simulink model "FixedWing_Model_nonlinearLQR_6_states"  (R2020b)
settings: Solver=VariableStepAuto  StartTime=0.0  StopTime=50  FixedStep=10^-4  RelTol=1e-7
values from neighbouring files (symbols this model uses):
  A_lat = [YB        Yp      -(u0-Yr)   g*cos(Theta0)   0;         A21       A22       A23        0             0;         A31       A32       A33        0             0;         0         1         0          0             0;         0         0         1          0             0]    [LQR_Dena_model_file_edited.m]
  A_long = [ Xu                    Xw              0              -g*cos(Theta0)            0;          Zu                    Zw              u0             -g*sin(Theta0)            0;          Mu+Mw_d*Zu            Mw+Mw_d*Zw      Mq+Mw_d*u0          0                    0;          0                     0               1                   0                    0;          -sin(Theta0)       -cos(Theta0)    ...(+51 chars)    [LQR_Dena_model_file_edited.m]
  b = 1.7    [LQR_Dena_model_file_edited.m]
  B_lat = [0        Ydr;        B21      B22;        B31      B32;        0        0;        0        0]    [LQR_Dena_model_file_edited.m]
  B_long = [ Xe         CXt;          Ze         0;          Me         0;          0          0;          0          0]    [LQR_Dena_model_file_edited.m]
  c = 0.28    [LQR_Dena_model_file_edited.m]
  C_lat = [0 0 0 1 0 ]    [LQR_Dena_model_file_edited.m]
  C_long = [0 0 0 1 0]    [LQR_Dena_model_file_edited.m]
  CL_aileron = 0.32935    [LQR_Dena_model_file_edited.m]
  CL_rudder = 0.003592    [LQR_Dena_model_file_edited.m]
  CLb = 0.029196    [LQR_Dena_model_file_edited.m]
  CLp = -0.44965    [LQR_Dena_model_file_edited.m]
  CLr = 0.0067709    [LQR_Dena_model_file_edited.m]
  CM_alpha = -0.1651    [LQR_Dena_model_file_edited.m]
  CM_alpha_dot = -6.5034    [LQR_Dena_model_file_edited.m]
  CMe = -1.3977    [LQR_Dena_model_file_edited.m]
  CMq = -11.7782    [LQR_Dena_model_file_edited.m]
  CMt = 0    [LQR_Dena_model_file_edited.m]
  CMu = 0.158*0    (= 0)    [LQR_Dena_model_file_edited.m]
  CN_aileron = 0.036215    [LQR_Dena_model_file_edited.m]
  CN_rudder = -0.045652    [LQR_Dena_model_file_edited.m]
  CNB = 0.066996    [LQR_Dena_model_file_edited.m]
  CNp = -0.030754    [LQR_Dena_model_file_edited.m]
  CNr = -0.064937    [LQR_Dena_model_file_edited.m]
  CX0 = -0.0094304    [LQR_Dena_model_file_edited.m]
  CX_alpha = (0.42565-0.21544)    (= 0.21021)    [LQR_Dena_model_file_edited.m]
  CXe = 0    [LQR_Dena_model_file_edited.m]
  CXt = 1    [LQR_Dena_model_file_edited.m]
  CXu = -(0.158*0)-0.0094304    (= -0.0094304)    [LQR_Dena_model_file_edited.m]
  CY_rudder = -0.10317    [LQR_Dena_model_file_edited.m]
  CYB = -0.16533    [LQR_Dena_model_file_edited.m]
  CYp = -0.00068802    [LQR_Dena_model_file_edited.m]
  CYr = 0.15502    [LQR_Dena_model_file_edited.m]
  CZ0 = -0.42565    [LQR_Dena_model_file_edited.m]
  CZ_alpha = -(4.8375+0.0094304)    (= -4.8469304)    [LQR_Dena_model_file_edited.m]
  CZ_alpha_dot = 1.3359    [LQR_Dena_model_file_edited.m]
  CZe = -0.56118    [LQR_Dena_model_file_edited.m]
  CZq = -7.3583    [LQR_Dena_model_file_edited.m]
  CZt = 0    [LQR_Dena_model_file_edited.m]
  CZu = -((0.052968^2)/(1-(0.052968)^2))*0.42565    (= -0.00119756738693)    [LQR_Dena_model_file_edited.m]
  d_aileron0 = 0    [LQR_Dena_model_file_edited.m]
  d_elevator0 = -0.6319*pi/180    (= -0.0110287355434)    [LQR_Dena_model_file_edited.m]
  D_long = zeros(5,2)    [LQR_Dena_model_file_edited.m]
  d_rudder0 = 0    [LQR_Dena_model_file_edited.m]
  d_Thrust0 = 5    [LQR_Dena_model_file_edited.m]
  e_longi = longd- [longi; 0]    [LQR_Dena_model_file_edited.m]
  Epsi0 = 0    [LQR_Dena_model_file_edited.m]
  Epsi_initial = Epsi0    (= 0)    [LQR_Dena_model_file_edited.m]
  g = 9.81    [LQR_Dena_model_file_edited.m]
  Hi = 120    [LQR_Dena_model_file_edited.m]
  Ix = 0.6465    [LQR_Dena_model_file_edited.m]
  Ixz = 0.0006584    [LQR_Dena_model_file_edited.m]
  Iy = 0.3048    [LQR_Dena_model_file_edited.m]
  Iz = 0.9359    [LQR_Dena_model_file_edited.m]
  K = K_long_hat(:,1:5)    [LQR_Dena_model_file_edited.m]
  K_lat_hat = lqr(A_lat_hat, B_lat_hat,Q_lat_hat,R_lat)    [LQR_Dena_model_file_edited.m]
  K_long = lqr(A_long, B_long,Q_long,R_long)    [LQR_Dena_model_file_edited.m]
  K_long_hat = lqr(A_long_hat, B_long_hat,Q_long_hat,R_long)    [LQR_Dena_model_file_edited.m]
  Ki = -K_long_hat(:,6)    [LQR_Dena_model_file_edited.m]
  lati = [ v_initial; p_initial; r_initial; Phi_initial; Epsi_initial]    [LQR_Dena_model_file_edited.m]
  longd = [u0; w0; q0; Theta0; Hi; 0]    [LQR_Dena_model_file_edited.m]
  longi = [ u_initial; w_initial; q_initial; Theta_initial; Ze0]    [LQR_Dena_model_file_edited.m]
  mass = 4    [LQR_Dena_model_file_edited.m]
  p0 = 0    [LQR_Dena_model_file_edited.m]
  p_initial = 0    [LQR_Dena_model_file_edited.m]
  Phi0 = 0    [LQR_Dena_model_file_edited.m]
  Phi_initial = Phi0    (= 0)    [LQR_Dena_model_file_edited.m]
  q0 = 0    [LQR_Dena_model_file_edited.m]
  q_initial = 0    [LQR_Dena_model_file_edited.m]
  r0 = 0    [LQR_Dena_model_file_edited.m]
  r_initial = 0    [LQR_Dena_model_file_edited.m]
  S = 0.471    [LQR_Dena_model_file_edited.m]
  Theta0 = 5.1*pi/180    (= 0.0890117918517)    [LQR_Dena_model_file_edited.m]
  Theta_initial = Theta0+(2*pi/180)    (= 0.123918376892)    [LQR_Dena_model_file_edited.m]
  u0 = sqrt(V0^2/(1+(tan(Theta0))^2))    [LQR_Dena_model_file_edited.m]
  u_initial = u0    [LQR_Dena_model_file_edited.m]
  v0 = 0    [LQR_Dena_model_file_edited.m]
  v_initial = v0    (= 0)    [LQR_Dena_model_file_edited.m]
  w0 = u0*tan(Theta0)    [LQR_Dena_model_file_edited.m]
  w_initial = w0    [LQR_Dena_model_file_edited.m]
  X0 = mass*g*sin(Theta0)    [LQR_Dena_model_file_edited.m]
  Xe0 = 0    [LQR_Dena_model_file_edited.m]
  Y0 = -mass*g*cos(Theta0)*sin(Phi0)    [LQR_Dena_model_file_edited.m]
  Ye0 = 0    [LQR_Dena_model_file_edited.m]
  Z0 = -mass*g*cos(Theta0)*cos(Phi0)    [LQR_Dena_model_file_edited.m]
  Ze0 = 120    [LQR_Dena_model_file_edited.m]
undefined symbols (not defined in the file or in its folder): A_hat, B_hat, C_hat, K_alt, K_e, Meu_e, use, W_e
libraries: simulink_extras x39, dspindex x3, aerolibatmos2 x1, aerolibutil x1, sharedtransform x1
(part 1 of 2)
settings Model: Creator=IT Solutions  LastModifiedBy=Roooooomaaaaaaaaaaaa
settings SolverCC: AlgebraicLoopSolver=LineSearch
settings DebuggingCC: UnconnectedInputMsg=none  UnconnectedOutputMsg=none  UnconnectedLineMsg=none  SFMachineParentedDataDiag=error

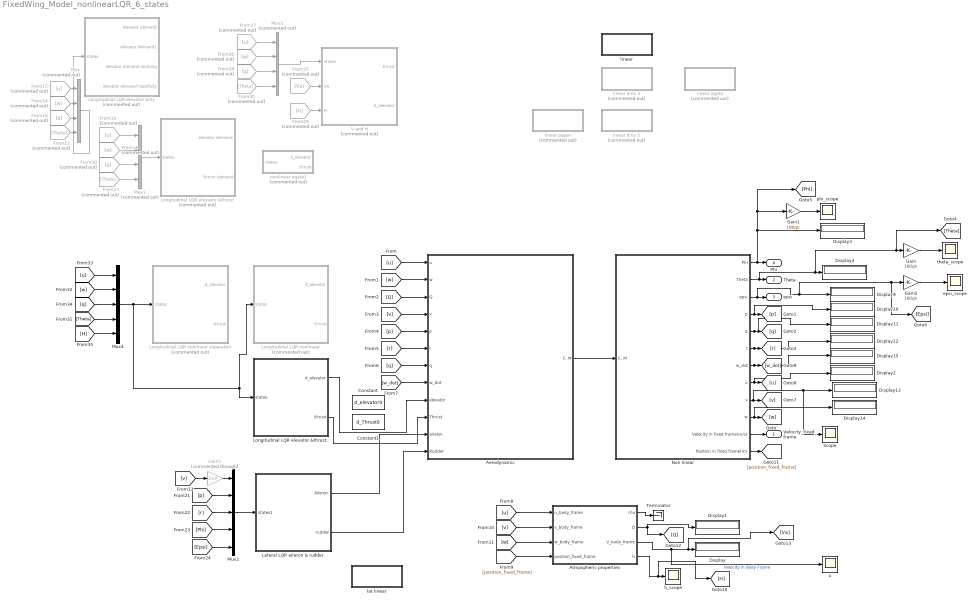
== system FixedWing_Model_nonlinearLQR_6_states ==
  "Aerodynamic " : Subsystem
  Atmpspheric properties : Subsystem
  Constant : Constant  Value=d_elevator0
  Constant1 : Constant  Value=d_Thrust0
  Display{,1..4,9..15} (12 alike) : Display
  From12 : From  Commented=on  GotoTag=Theta
  From14 : From  Commented=on  GotoTag=w
  From15 : From  Commented=on  GotoTag=u
  From16 : From  Commented=on  GotoTag=q
  From17 : From  Commented=on  GotoTag=Theta
  From18 : From  Commented=on  GotoTag=w
  From19 : From  Commented=on  GotoTag=u
  From20 : From  Commented=on  GotoTag=q
  From25 : From  Commented=on  GotoTag=Va
  From26 : From  Commented=on  GotoTag=w
  From27 : From  Commented=on  GotoTag=u
  From28 : From  Commented=on  GotoTag=q
  From29 : From  Commented=on  GotoTag=H
  From30 : From  Commented=on  GotoTag=Theta
  Gain : Gain  Gain=180/pi
  Gain1 : Gain  Gain=180/pi
  Gain2 : Gain  Gain=180/pi
  Gain3 : Gain  Commented=through  Gain=1/u0
  Lateral LQR aileron & rudder : Subsystem
  Longitudinal LQR elevator &thrust : Subsystem  Commented=on
  Longitudinal LQR elevator &thrust. : Subsystem
  Longitudinal LQR elevator only : Subsystem  Commented=on
  Longitudinal LQR nonlinear : Subsystem  Commented=on
  Longitudinal LQR nonlinear seperated : Subsystem  Commented=on
  Mux : Mux  Commented=on
  Mux1 : Mux  Commented=on
  Mux2 : Mux  Inputs=5
  Mux3 : Mux  Commented=on
  Mux4 : Mux  Inputs=5
  Non linear : Subsystem
  Scope : Scope
  Terminator : Terminator
  V and H : Subsystem  Commented=on
  epsi_scope : Scope
  h_scope : Scope
  lat linear : Subsystem
  linear : Subsystem
  linear dina 4 : Subsystem  Commented=on
  linear dina 5 : Subsystem  Commented=on
  linear ogata : Subsystem  Commented=on
  linear paper : Subsystem  Commented=on
  nonlinear ogata1 : Subsystem  Commented=on
  phi_scope : Scope
  theta_scope : Scope
  u : Scope
  Velocity_fixed_frame : Outport
  Theta : Outport  Port=2
  epsi : Outport  Port=3
  Phi : Outport  Port=4
  wires:
  [u] -> "Aerodynamic "/1(u)
  [w] -> "Aerodynamic "/2(w)
  [v] -> "Aerodynamic "/4(v)
  [p] -> "Aerodynamic "/5(p)
  [r] -> "Aerodynamic "/6(r)
  [q] -> "Aerodynamic "/7(q)
  [w_dot] -> "Aerodynamic "/8(w_dot)
  Non linear/4(p) -> Display10/1, [p]
  Non linear/5(q) -> Display11/1, [q]
  Non linear/6(r) -> Display12/1, [r]
  Non linear/1(Phi) -> Display3/1, Gain1/1, [Phi], Phi/1
  Non linear/3(epsi) -> Gain2/1, [Epsi], Display9/1, epsi/1
  Non linear/7(w_dot) -> Display15/1, [w_dot]
  Non linear/8(u) -> Display2/1, [u]
  Non linear/9(v) -> Scope/1, Display13/1, [v]
  Non linear/10(w) -> Display14/1, [w]
  Non linear/11(Velocity in fixed frame(m/s)) -> Velocity_fixed_frame/1
  Non linear/12(Position in fixed frame(m)) -> [position_fixed_frame]
  [position_fixed_frame] -> Atmpspheric properties/4(position_fixed_frame)
  Atmpspheric properties/2(Q) -> [Q], Display1/1
  Atmpspheric properties/1(rho) -> Terminator/1
  [u] -> Atmpspheric properties/1(u_body_frame)
  [v] -> Atmpspheric properties/2(v_body_frame)
  [w] -> Atmpspheric properties/3(w_body_frame)
  Atmpspheric properties/3(V_body_frame) -> u/1, [Va], Display/1  "Velocity in Body Frame"
  Non linear/2(Theta) -> [Theta], Gain/1, Display4/1, Theta/1
  [Q] -> "Aerodynamic "/3(Q)
  "Aerodynamic "/1("F, M") -> Non linear/1("F, M")
  Gain/1 -> theta_scope/1
  Atmpspheric properties/4(h) -> [H], h_scope/1
  Gain1/1 -> phi_scope/1
  Gain2/1 -> epsi_scope/1
  From12/1 -> Mux/4
  From16/1 -> Mux/3
  From14/1 -> Mux/2
  From15/1 -> Mux/1
  Mux/1 -> Longitudinal LQR elevator only/1(states)
  From20/1 -> Mux1/3
  From17/1 -> Mux1/4
  Mux1/1 -> Longitudinal LQR elevator &thrust/1(states)
  From18/1 -> Mux1/2
  From19/1 -> Mux1/1
  Mux2/1 -> Lateral LQR aileron & rudder/1(states1)
  [p] -> Mux2/2
  [r] -> Mux2/3
  [Phi] -> Mux2/4
  [v] -> Gain3/1
  From26/1 -> Mux3/2
  From30/1 -> Mux3/4
  From27/1 -> Mux3/1
  From28/1 -> Mux3/3
  Mux3/1 -> V and H/1(states)
  From25/1 -> V and H/2(Va)
  From29/1 -> V and H/3(H)
  [w] -> Mux4/2
  [Theta] -> Mux4/4
  [q] -> Mux4/3
  [u] -> Mux4/1
  Mux4/1 -> Longitudinal LQR nonlinear/1(states), Longitudinal LQR elevator &thrust./1(states), Longitudinal LQR nonlinear seperated/1(states)
  [H] -> Mux4/5
  Lateral LQR aileron & rudder/1(Aileron) -> "Aerodynamic "/11(airelon)
  Lateral LQR aileron & rudder/2(rudder) -> "Aerodynamic "/12(Rudder)
  [Epsi] -> Mux2/5
  Gain3/1 -> Mux2/1
  Longitudinal LQR elevator &thrust./1(d_elevator) -> "Aerodynamic "/9(elevator)
  Longitudinal LQR elevator &thrust./2(thrust) -> "Aerodynamic "/10(Thrust)

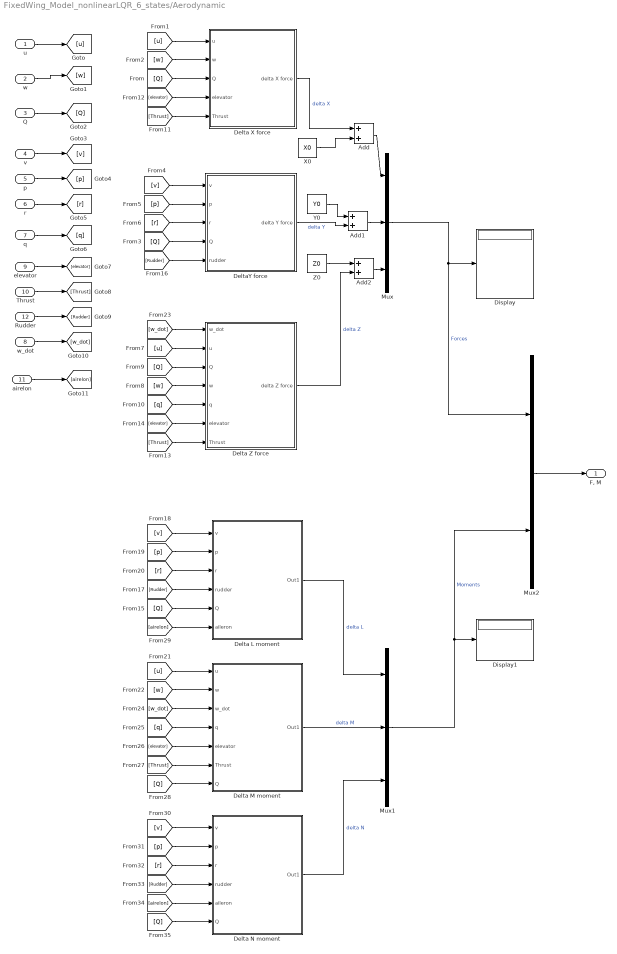
== system FixedWing_Model_nonlinearLQR_6_states/Aerodynamic  ==
  u : Inport
  w : Inport  Port=2
  Q : Inport  Port=3
  v : Inport  Port=4
  p : Inport  Port=5
  r : Inport  Port=6
  q : Inport  Port=7
  w_dot : Inport  Port=8
  elevator : Inport  Port=9
  Thrust : Inport  Port=10
  airelon : Inport  Port=11
  Rudder : Inport  Port=12
  Add : Sum
  Add1 : Sum
  Add2 : Sum
  Delta L moment : Subsystem
  Delta M moment : Subsystem
  Delta N moment : Subsystem
  Delta X force : Subsystem
  Delta Z force : Subsystem
  DeltaY force : Subsystem
  Display : Display
      settings: Decimation=3
  Display1 : Display
      settings: Decimation=3
  Mux : Mux  Inputs=3
  Mux1 : Mux  Inputs=3
  Mux2 : Mux  Inputs=2
  X0 : Constant  Value=X0
  Y0 : Constant  Value=Y0
  Z0 : Constant  Value=Z0
  "F, M" : Outport
  wires:
  Mux/1 -> Mux2/1, Display/1  "Forces"
  Mux1/1 -> Mux2/2, Display1/1  "Moments"
  DeltaY force/1(delta Y force) -> Add1/2  "delta Y"
  Delta L moment/1(Out1) -> Mux1/1  "delta L"
  Mux2/1 -> "F, M"/1
  Q/1 -> [Q]
  w/1 -> [w]
  u/1 -> [u]
  Delta N moment/1(Out1) -> Mux1/3  "delta N"
  [Q] -> DeltaY force/4(Q)
  [Rudder] -> DeltaY force/5(rudder)
  v/1 -> [v]
  p/1 -> [p]
  r/1 -> [r]
  [v] -> DeltaY force/1(v)
  [p] -> DeltaY force/2(p)
  [r] -> DeltaY force/3(r)
  q/1 -> [q]
  elevator/1 -> [elevator]
  Thrust/1 -> [Thrust]
  [Q] -> Delta L moment/5(Q)
  Rudder/1 -> [Rudder]
  [Rudder] -> Delta L moment/4(rudder)
  [v] -> Delta L moment/1(v)
  [p] -> Delta L moment/2(p)
  [r] -> Delta L moment/3(r)
  w_dot/1 -> [w_dot]
  airelon/1 -> [airelon]
  [airelon] -> Delta L moment/6(aileron)
  [v] -> Delta N moment/1(v)
  [p] -> Delta N moment/2(p)
  [r] -> Delta N moment/3(r)
  [Rudder] -> Delta N moment/4(rudder)
  [airelon] -> Delta N moment/5(aileron)
  [Q] -> Delta N moment/6(Q)
  X0/1 -> Add/2
  Y0/1 -> Add1/1
  Z0/1 -> Add2/1
  Add/1 -> Mux/1
  Add1/1 -> Mux/2
  Add2/1 -> Mux/3
  [u] -> Delta Z force/2(u)
  [w] -> Delta Z force/4(w)
  [w_dot] -> Delta Z force/1(w_dot)
  Delta Z force/1(delta Z force) -> Add2/2  "delta Z"
  [Q] -> Delta Z force/3(Q)
  [q] -> Delta Z force/5(q)
  [elevator] -> Delta Z force/6(elevator)
  [w] -> Delta X force/2(w)
  [elevator] -> Delta X force/4(elevator)
  [Q] -> Delta X force/3(Q)
  [u] -> Delta X force/1(u)
  Delta X force/1(delta X force) -> Add/1  "delta X"
  [q] -> Delta M moment/4(q)
  Delta M moment/1(Out1) -> Mux1/2  "delta M"
  [elevator] -> Delta M moment/5(elevator)
  [Q] -> Delta M moment/7(Q)
  [Thrust] -> Delta M moment/6(Thrust)
  [w] -> Delta M moment/2(w)
  [w_dot] -> Delta M moment/3(w_dot)
  [u] -> Delta M moment/1(u)
  [Thrust] -> Delta X force/5(Thrust)
  [Thrust] -> Delta Z force/7(Thrust)

== system FixedWing_Model_nonlinearLQR_6_states/Atmpspheric properties ==
  u_body_frame : Inport
  v_body_frame : Inport  Port=2
  w_body_frame : Inport  Port=3
  position_fixed_frame : Inport  Port=4
  Add : Sum  Inputs=+++
  Demux : Demux  Outputs=3
  Display : Display
  Gain : Gain  Gain=1/2
  ISA Atmosphere Model : aerolibatmos2/ISA Atmosphere Model  custom=off  g=9.80665  gamma=1.4  R=287.0531  L=0.0065  h_trop=11000  h_strat=20000  rho0=1.225  P0=101325  T0=288.15  h0=0
  Product : Product
  Scope : Scope
  Sqrt : Sqrt  SaturateOnIntegerOverflow=on
  Square : Math  Operator=square  SaturateOnIntegerOverflow=on
  Square1 : Math  Operator=square  SaturateOnIntegerOverflow=on
  Square2 : Math  Operator=square  SaturateOnIntegerOverflow=on
  Terminator : Terminator
  Terminator1 : Terminator
  rho : Outport
  Q : Outport  Port=2
  V_body_frame : Outport  Port=3
  h : Outport  Port=4
  wires:
  position_fixed_frame/1 -> Demux/1
  Demux/1 -> Terminator/1
  Demux/2 -> Terminator1/1
  Demux/3 -> Scope/1, h/1, ISA Atmosphere Model/1
  ISA Atmosphere Model/4 -> [rho], rho/1
  Square/1 -> Add/1
  Square1/1 -> Add/2
  Square2/1 -> Add/3
  Add/1 -> Sqrt/1, Gain/1
  Gain/1 -> Product/2
  [rho] -> Product/1
  Product/1 -> Q/1
  u_body_frame/1 -> Square/1
  v_body_frame/1 -> Square1/1
  w_body_frame/1 -> Square2/1
  Sqrt/1 -> Display/1, V_body_frame/1

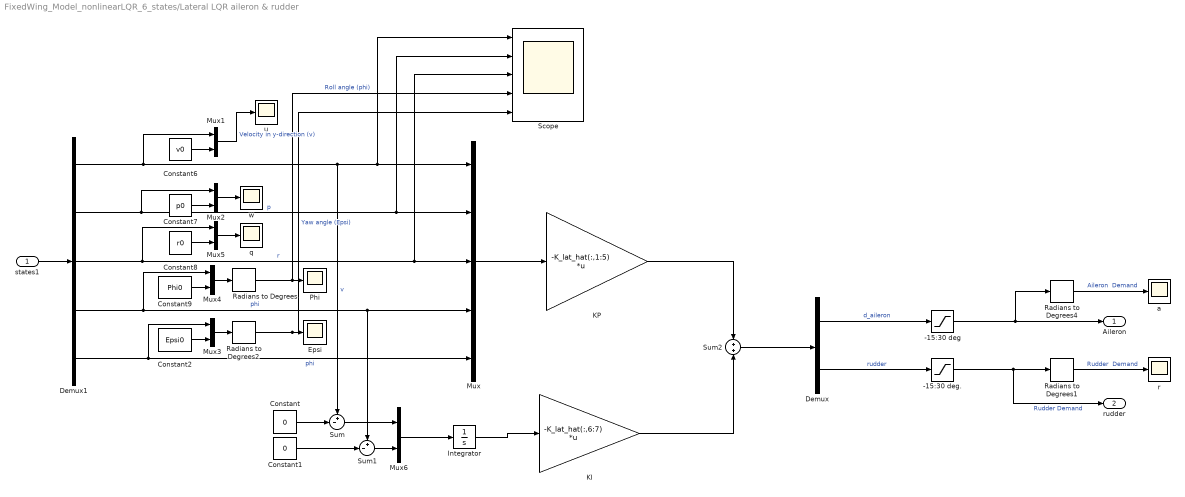
== system FixedWing_Model_nonlinearLQR_6_states/Lateral LQR aileron & rudder ==
  states1 : Inport
  -15:30 deg : Saturate  UpperLimit=30*pi/180  LowerLimit=-15*pi/180
  -15:30 deg. : Saturate  UpperLimit=30*pi/180  LowerLimit=-15*pi/180
  Constant : Constant  Value=0
  Constant1 : Constant  Value=0
  Constant2 : Constant  Value=Epsi0
  Constant6 : Constant  Value=v0
  Constant7 : Constant  Value=p0
  Constant8 : Constant  Value=r0
  Constant9 : Constant  Value=Phi0
  Demux : Demux  Outputs=2
  Demux1 : Demux  Outputs=5
  Epsi : Scope
  Integrator : Integrator
  KI : Gain  Gain=-K_lat_hat(:,6:7)  Multiplication=Matrix(K*u)
  KP : Gain  Gain=-K_lat_hat(:,1:5)  Multiplication=Matrix(K*u)
  Mux : Mux  Inputs=5
  Mux{1..6} (6 alike) : Mux  Inputs=2
  Phi : Scope
  Radians to Degrees{,1..2,4} (4 alike) : simulink_extras/Transformations/Radians to Degrees
  Scope : Scope  NumInputPorts=5
  Sum : Sum  Inputs=+-|
  Sum1 : Sum  Inputs=+-|
  Sum2 : Sum  Inputs=+|+
  a : Scope
  q : Scope
  r : Scope
  u : Scope
  w : Scope
  Aileron : Outport
  rudder : Outport  Port=2
  wires:
  Sum2/1 -> Demux/1
  Demux1/2 -> Scope/2, Mux/2, Mux2/1  "p"
  Constant9/1 -> Mux4/2
  Mux1/1 -> u/1  "Velocity in y-direction (v)"
  Constant/1 -> Sum/2
  Mux/1 -> KP/1
  Demux1/4 -> Mux4/1, Sum1/1, Mux/4  "phi"
  Constant6/1 -> Mux1/2
  Integrator/1 -> KI/1
  KP/1 -> Sum2/1
  Mux4/1 -> Radians to Degrees/1
  Mux6/1 -> Integrator/1
  Sum1/1 -> Mux6/2
  Mux5/1 -> q/1
  Sum/1 -> Mux6/1
  Constant8/1 -> Mux5/2
  Demux1/1 -> Scope/1, Mux/1, Sum/1, Mux1/1  "v"
  Constant7/1 -> Mux2/2
  KI/1 -> Sum2/2
  Radians to Degrees/1 -> Scope/4, Phi/1  "Roll angle (phi)"
  Mux2/1 -> w/1
  Radians to Degrees4/1 -> a/1  "Aileron  Demand"
  Demux/2 -> -15:30 deg./1  "rudder"
  Demux/1 -> -15:30 deg/1  "d_aileron"
  states1/1 -> Demux1/1
  Constant1/1 -> Sum1/2
  -15:30 deg/1 -> Radians to Degrees4/1, Aileron/1
  Demux1/3 -> Scope/3, Mux/3, Mux5/1  "r"
  -15:30 deg./1 -> Radians to Degrees1/1, rudder/1  "Rudder Demand"
  Radians to Degrees1/1 -> r/1  "Rudder  Demand"
  Radians to Degrees2/1 -> Scope/5, Epsi/1  "Yaw angle (Epsi)"
  Mux3/1 -> Radians to Degrees2/1
  Demux1/5 -> Mux3/1, Mux/5  "phi"
  Constant2/1 -> Mux3/2

== system FixedWing_Model_nonlinearLQR_6_states/Longitudinal LQR elevator &thrust ==
  states : Inport
  all system : Subsystem
  "elevator demand " : Outport
  thrust demand : Outport  Port=2
  wires:
  all system/1(d_elevator) -> "elevator demand "/1
  states/1 -> all system/1(states)
  all system/2(thrust) -> thrust demand/1

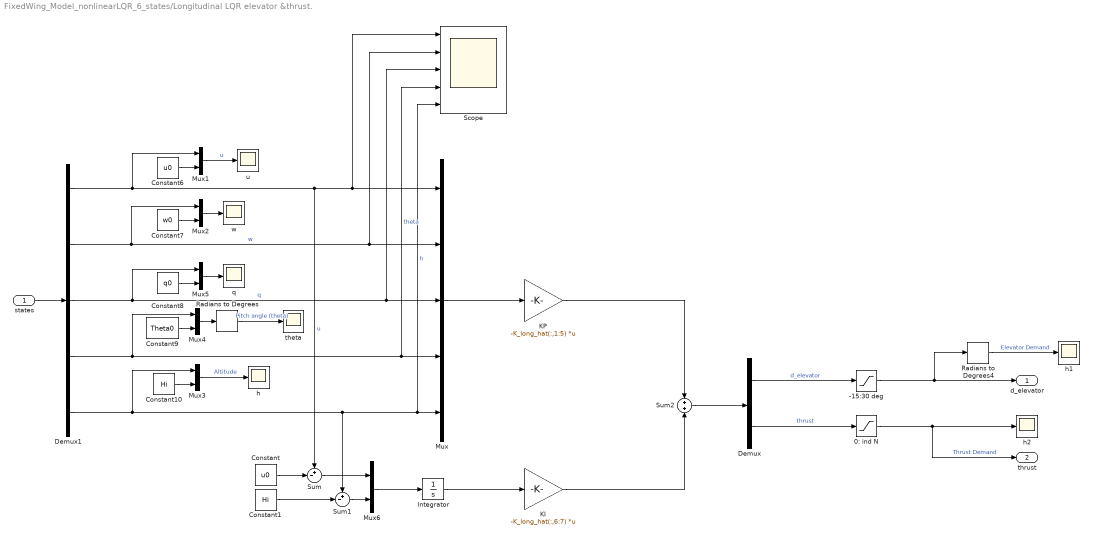
== system FixedWing_Model_nonlinearLQR_6_states/Longitudinal LQR elevator &thrust. ==
  states : Inport
  -15:30 deg : Saturate  UpperLimit=30*pi/180  LowerLimit=-15*pi/180
  0: ind N : Saturate  UpperLimit=inf  LowerLimit=0
  Constant : Constant  Value=u0
  Constant1 : Constant  Value=Hi
  Constant10 : Constant  Value=Hi
  Constant6 : Constant  Value=u0
  Constant7 : Constant  Value=w0
  Constant8 : Constant  Value=q0
  Constant9 : Constant  Value=Theta0
  Demux : Demux  Outputs=2
  Demux1 : Demux  Outputs=5
  Integrator : Integrator
  KI : Gain  Gain=-K_long_hat(:,6:7)  Multiplication=Matrix(K*u)
  KP : Gain  Gain=-K_long_hat(:,1:5)  Multiplication=Matrix(K*u)
  Mux : Mux  Inputs=5
  Mux{1..6} (6 alike) : Mux  Inputs=2
  Radians to Degrees : simulink_extras/Transformations/Radians to Degrees
  Radians to Degrees4 : simulink_extras/Transformations/Radians to Degrees
  Scope : Scope  NumInputPorts=5
  Sum : Sum  Inputs=+-|
  Sum1 : Sum  Inputs=+-|
  Sum2 : Sum  Inputs=+|+
  h : Scope
  h1 : Scope
  h2 : Scope
  q : Scope
  theta : Scope
  u : Scope
  w : Scope
  d_elevator : Outport
  thrust : Outport  Port=2
  wires:
  Radians to Degrees4/1 -> h1/1  "Elevator Demand"
  Demux/2 -> 0: ind N/1  "thrust"
  Demux/1 -> -15:30 deg/1  "d_elevator"
  KP/1 -> Sum2/1
  -15:30 deg/1 -> Radians to Degrees4/1, d_elevator/1
  0: ind N/1 -> h2/1, thrust/1  "Thrust Demand"
  states/1 -> Demux1/1
  Mux5/1 -> q/1
  Sum/1 -> Mux6/1
  Sum1/1 -> Mux6/2
  Demux1/5 -> Scope/5, Mux/5, Sum1/1, Mux3/1  "h"
  Mux4/1 -> Radians to Degrees/1
  Mux6/1 -> Integrator/1
  Constant6/1 -> Mux1/2
  Integrator/1 -> KI/1
  Demux1/4 -> Scope/4, Mux/4, Mux4/1  "theta"
  Mux/1 -> KP/1
  Mux2/1 -> w/1
  Demux1/3 -> Scope/3, Mux/3, Mux5/1  "q"
  Constant/1 -> Sum/2
  Mux1/1 -> u/1  "u"
  Constant10/1 -> Mux3/2
  Constant9/1 -> Mux4/2
  Radians to Degrees/1 -> theta/1  "Pitch angle (theta)"
  Demux1/2 -> Scope/2, Mux/2, Mux2/1  "w"
  Demux1/1 -> Scope/1, Mux/1, Sum/1, Mux1/1  "u"
  KI/1 -> Sum2/2
  Constant7/1 -> Mux2/2
  Mux3/1 -> h/1  "Altitude"
  Constant1/1 -> Sum1/2
  Constant8/1 -> Mux5/2
  Sum2/1 -> Demux/1

== system FixedWing_Model_nonlinearLQR_6_states/Longitudinal LQR elevator only ==
  states : Inport
  Actual theta2 : Scope
  Demux1 : Demux
  Radians to Degrees6 : simulink_extras/Transformations/Radians to Degrees
  Servo2 : TransferFcn  Commented=on  Numerator=[K_e]  Denominator=[W_e^(-2) (2*Meu_e/W_e) 1]
  all system : Subsystem
  states from ss : Subsystem  Commented=on
  theta from ss : Subsystem  Commented=on
  theta system only : Subsystem
  elevator demand : Outport
  elevator demand1 : Outport  Port=2
  elevator demand working : Outport  Port=3
  elevator demand hopefully : Outport  Port=4
  wires:
  Radians to Degrees6/1 -> Actual theta2/1
  Demux1/4 -> Radians to Degrees6/1, [theta]
  theta system only/1(d_elevator) -> elevator demand working/1
  [theta] -> theta system only/1(theta)
  all system/1(d_elevator) -> elevator demand hopefully/1
  states/1 -> Demux1/1, all system/1(states)
  theta from ss/1(elevator demand) -> elevator demand/1
  states from ss/1(elevator demand1) -> elevator demand1/1

== system FixedWing_Model_nonlinearLQR_6_states/Longitudinal LQR nonlinear ==
  states : Inport
  Constant1 : Constant  Value=d_elevator0
  Constant2 : Constant  Value=d_Thrust0
  Demux : Demux  Outputs=2
  Gain : Gain
  Gain1 : Gain
  K_LQR : Gain  Gain=K_long_hat  Multiplication=Matrix(K*u)
  Radians to Degrees4 : simulink_extras/Transformations/Radians to Degrees
  Sum1 : Sum  Inputs=|++
  Sum2 : Sum  Inputs=|++
  Thrust : Scope
  elevator2 : Scope
  states' error : Subsystem
  d_elevator : Outport
  thrust : Outport  Port=2
  wires:
  Demux/2 -> Sum2/1
  Demux/1 -> Sum1/1
  Sum2/1 -> Gain1/1, Thrust/1  "thrust"
  Sum1/1 -> Gain/1, Radians to Degrees4/1  "d_elevator"
  states' error/1(states' error) -> K_LQR/1
  Radians to Degrees4/1 -> elevator2/1
  states/1 -> states' error/1(In1)
  K_LQR/1 -> Demux/1
  Constant1/1 -> Sum1/2
  Constant2/1 -> Sum2/2
  Gain/1 -> d_elevator/1
  Gain1/1 -> thrust/1

== system FixedWing_Model_nonlinearLQR_6_states/Longitudinal LQR nonlinear seperated ==
  states : Inport
  Constant1 : Constant  Value=d_elevator0
  Constant2 : Constant  Value=d_Thrust0
  Demux : Demux  Outputs=2
  Gain : Gain  Gain=K  Multiplication=Matrix(K*u)
  Gain1 : Gain  Gain=Ki  Multiplication=Matrix(K*u)
  Integrator : Integrator
  Radians to Degrees4 : simulink_extras/Transformations/Radians to Degrees
  Sum1 : Sum  Inputs=|++
  Sum2 : Sum  Inputs=|++
  Sum3 : Sum  Inputs=|-+
  Thrust : Scope
  elevator2 : Scope
  theta' error : Subsystem
  d_elevator : Outport
  thrust : Outport  Port=2
  wires:
  Demux/2 -> Sum2/1
  Demux/1 -> Sum1/1
  Sum2/1 -> thrust/1, Thrust/1  "thrust"
  Sum1/1 -> d_elevator/1, Radians to Degrees4/1  "d_elevator"
  Radians to Degrees4/1 -> elevator2/1
  states/1 -> Gain/1, theta' error/1(states)
  Constant1/1 -> Sum1/2
  Constant2/1 -> Sum2/2
  Gain/1 -> Sum3/1
  Integrator/1 -> Gain1/1
  Gain1/1 -> Sum3/2
  theta' error/1(theta' error) -> Integrator/1
  Sum3/1 -> Demux/1  "d_elevator"

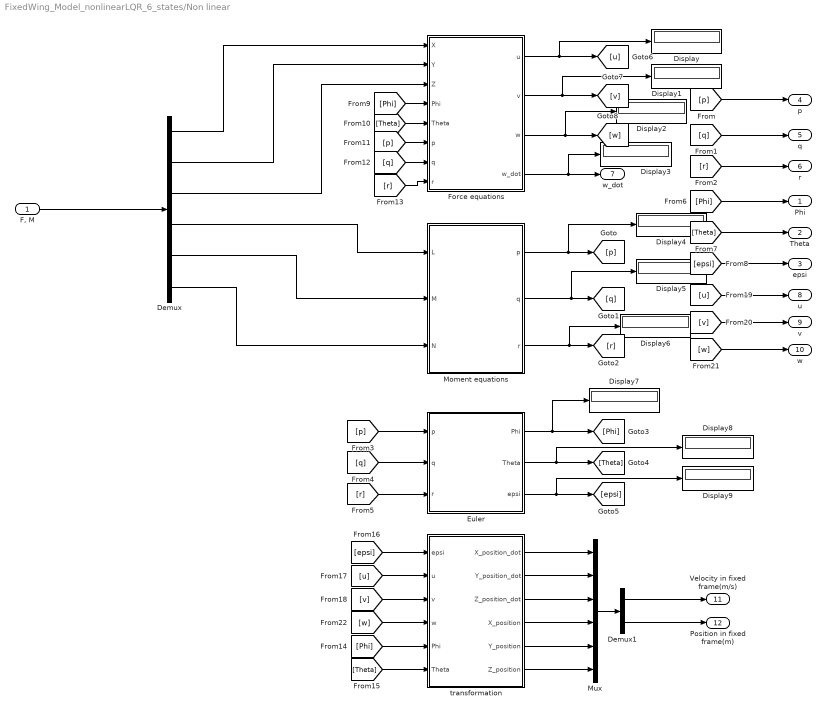
== system FixedWing_Model_nonlinearLQR_6_states/Non linear ==
  "F, M" : Inport
  Demux : Demux  Outputs=6
  Demux1 : Demux  Outputs=2
  Display{,1..9} (10 alike) : Display
  Euler : Subsystem
  Force equations : Subsystem
  Moment equations : Subsystem
  Mux : Mux  Inputs=6
  transformation : Subsystem
  Phi : Outport
  Theta : Outport  Port=2
  epsi : Outport  Port=3
  p : Outport  Port=4
  q : Outport  Port=5
  r : Outport  Port=6
  w_dot : Outport  Port=7
  u : Outport  Port=8
  v : Outport  Port=9
  w : Outport  Port=10
  Velocity in fixed frame(m/s) : Outport  Port=11
  Position in fixed frame(m) : Outport  Port=12
  wires:
  "F, M"/1 -> Demux/1
  Demux/2 -> Force equations/2(Y)
  Demux/4 -> Moment equations/1(L)
  Demux/3 -> Force equations/3(Z)
  Demux/1 -> Force equations/1(X)
  Force equations/1(u) -> Display/1, [u]
  Force equations/2(v) -> Display1/1, [v]
  Force equations/3(w) -> Display2/1, [w]
  [p] -> p/1
  [r] -> r/1
  [q] -> q/1
  Moment equations/2(q) -> Display5/1, [q]
  Moment equations/1(p) -> Display4/1, [p]
  Moment equations/3(r) -> Display6/1, [r]
  Demux/5 -> Moment equations/2(M)
  Demux/6 -> Moment equations/3(N)
  [q] -> Euler/2(q)
  [p] -> Euler/1(p)
  [r] -> Euler/3(r)
  [Phi] -> Phi/1
  [Theta] -> Theta/1
  [epsi] -> epsi/1
  Euler/1(Phi) -> Display7/1, [Phi]
  Euler/2(Theta) -> Display8/1, [Theta]
  Euler/3(epsi) -> Display9/1, [epsi]
  [Phi] -> Force equations/4(Phi)
  [Theta] -> Force equations/5(Theta)
  [p] -> Force equations/6(p)
  [q] -> Force equations/7(q)
  [r] -> Force equations/8(r)
  Force equations/4(w_dot) -> Display3/1, w_dot/1
  [u] -> u/1
  [v] -> v/1
  [w] -> w/1
  [Theta] -> transformation/6(Theta)
  [v] -> transformation/3(v)
  [u] -> transformation/2(u)
  [Phi] -> transformation/5(Phi)
  [epsi] -> transformation/1(epsi)
  [w] -> transformation/4(w)
  transformation/1(X_position_dot) -> Mux/1
  transformation/2(Y_position_dot) -> Mux/2
  transformation/3(Z_position_dot) -> Mux/3
  transformation/4(X_position) -> Mux/4
  transformation/5(Y_position) -> Mux/5
  transformation/6(Z_position) -> Mux/6
  Mux/1 -> Demux1/1
  Demux1/1 -> Velocity in fixed frame(m/s)/1
  Demux1/2 -> Position in fixed frame(m)/1

== system FixedWing_Model_nonlinearLQR_6_states/V and H ==
  states : Inport
  Va : Inport  Port=2
  H : Inport  Port=3
  Actual theta : Scope
  Constant : Constant  Value=120
  Constant1 : Constant  Value=d_elevator0
  Constant2 : Constant  Value=d_Thrust0
  Constant3 : Constant  Value=0
  Constant4 : Constant  Value=0
  Constant5 : Constant  Value=K_alt
  Demux : Demux  Outputs=2
  Derivative : Derivative
  Derivative1 : Derivative
  Gain1 : Gain
  Gain2 : Gain
  K_LQR : Gain  Gain=K_long  Multiplication=Matrix(K*u)
  MatrixMultiply : Product  Inputs=**  Multiplication=Matrix(*)
  Mux : Mux  Inputs=3
  Radians to Degrees4 : simulink_extras/Transformations/Radians to Degrees
  Sum1 : Sum  Inputs=|++
  Sum2 : Sum  Inputs=|++
  Sum3 : Sum  Inputs=|-+
  Sum4 : Sum  Inputs=|-+
  Sum5 : Sum  Inputs=|-+
  Thrust : Scope
  elevator2 : Scope
  states' error : Subsystem
  thrust : Outport
  d_elevator : Outport  Port=2
  wires:
  states' error/1(theta in degrees) -> Actual theta/1
  Gain1/1 -> thrust/1  "thrust"
  Sum2/1 -> Thrust/1, Gain1/1
  Demux/2 -> Sum2/1
  states/1 -> states' error/1(In1)
  states' error/2(states' error) -> K_LQR/1
  Constant2/1 -> Sum2/2
  K_LQR/1 -> Demux/1
  Constant1/1 -> Sum1/2
  Sum1/1 -> Gain2/1, Radians to Degrees4/1
  MatrixMultiply/1 -> Sum1/1
  Gain2/1 -> d_elevator/1  "d_elevator"
  Radians to Degrees4/1 -> elevator2/1
  Constant/1 -> Sum5/2
  H/1 -> Derivative/1, Sum5/1
  Derivative/1 -> Sum3/1, Derivative1/1
  Constant3/1 -> Sum3/2
  Constant4/1 -> Sum4/2
  Derivative1/1 -> Sum4/1
  Sum5/1 -> Mux/1  "error q"
  Sum3/1 -> Mux/2  "error q"
  Sum4/1 -> Mux/3  "error q"
  Mux/1 -> MatrixMultiply/1
  Constant5/1 -> MatrixMultiply/2

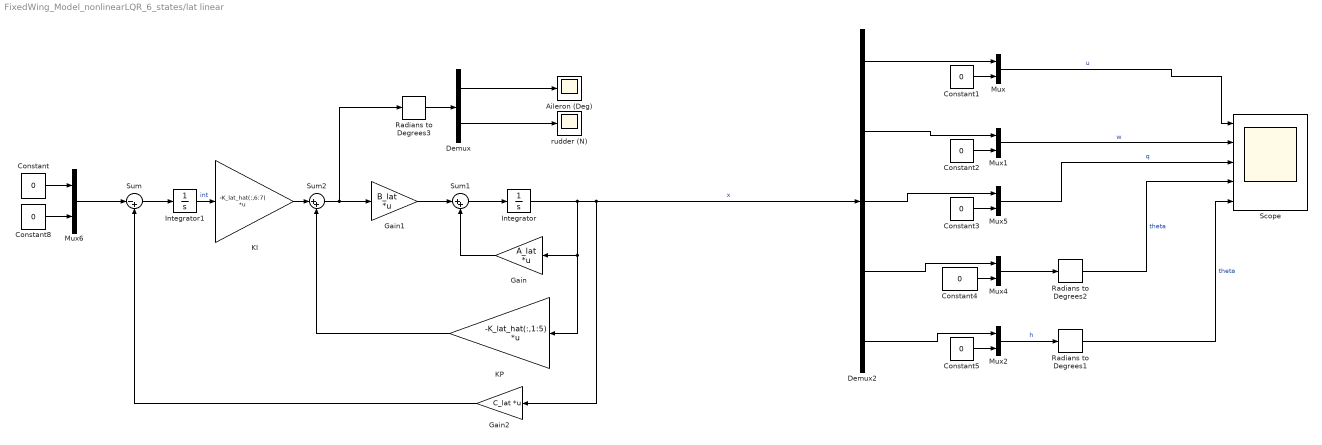
== system FixedWing_Model_nonlinearLQR_6_states/lat linear ==
  Aileron (Deg) : Scope
  Constant{,1..5,8} (7 alike) : Constant  Value=0
  Demux : Demux  Outputs=2
  Demux2 : Demux  Outputs=5
  Gain : Gain  Gain=A_lat  Multiplication=Matrix(K*u)
  Gain1 : Gain  Gain=B_lat  Multiplication=Matrix(K*u)
  Gain2 : Gain  Gain=C_lat  Multiplication=Matrix(K*u)
  Integrator : Integrator  InitialCondition=lati
  Integrator1 : Integrator
  KI : Gain  Gain=-K_lat_hat(:,6:7)  Multiplication=Matrix(K*u)
  KP : Gain  Gain=-K_lat_hat(:,1:5)  Multiplication=Matrix(K*u)
  Mux{,1..2,4..6} (6 alike) : Mux  Inputs=2
  Radians to Degrees1 : simulink_extras/Transformations/Radians to Degrees
  Radians to Degrees2 : simulink_extras/Transformations/Radians to Degrees
  Radians to Degrees3 : simulink_extras/Transformations/Radians to Degrees
  Scope : Scope  NumInputPorts=5
  Sum : Sum  Inputs=|-+
  Sum1 : Sum  Inputs=|++
  Sum2 : Sum  Inputs=|++
  rudder (N) : Scope
  wires:
  Sum1/1 -> Integrator/1
  Integrator/1 -> Demux2/1, Gain2/1, Gain/1, KP/1  "x"
  Gain/1 -> Sum1/2
  Gain1/1 -> Sum1/1
  Radians to Degrees2/1 -> Scope/4  "theta"
  Demux/1 -> Aileron (Deg)/1
  Demux/2 -> rudder (N)/1
  Mux/1 -> Scope/1  "u"
  Mux1/1 -> Scope/2  "w"
  Mux5/1 -> Scope/3  "q"
  Mux4/1 -> Radians to Degrees2/1
  Mux2/1 -> Radians to Degrees1/1  "h"
  Constant1/1 -> Mux/2
  Demux2/1 -> Mux/1
  Constant2/1 -> Mux1/2
  Constant3/1 -> Mux5/2
  Constant4/1 -> Mux4/2
  Constant5/1 -> Mux2/2
  Demux2/5 -> Mux2/1
  Demux2/4 -> Mux4/1
  Demux2/2 -> Mux1/1
  Demux2/3 -> Mux5/1
  Sum2/1 -> Radians to Degrees3/1, Gain1/1
  KP/1 -> Sum2/2
  Constant/1 -> Mux6/1
  Constant8/1 -> Mux6/2
  Sum/1 -> Integrator1/1
  KI/1 -> Sum2/1
  Mux6/1 -> Sum/1
  Gain2/1 -> Sum/2
  Integrator1/1 -> KI/1  "int"
  Radians to Degrees3/1 -> Demux/1
  Radians to Degrees1/1 -> Scope/5  "theta"

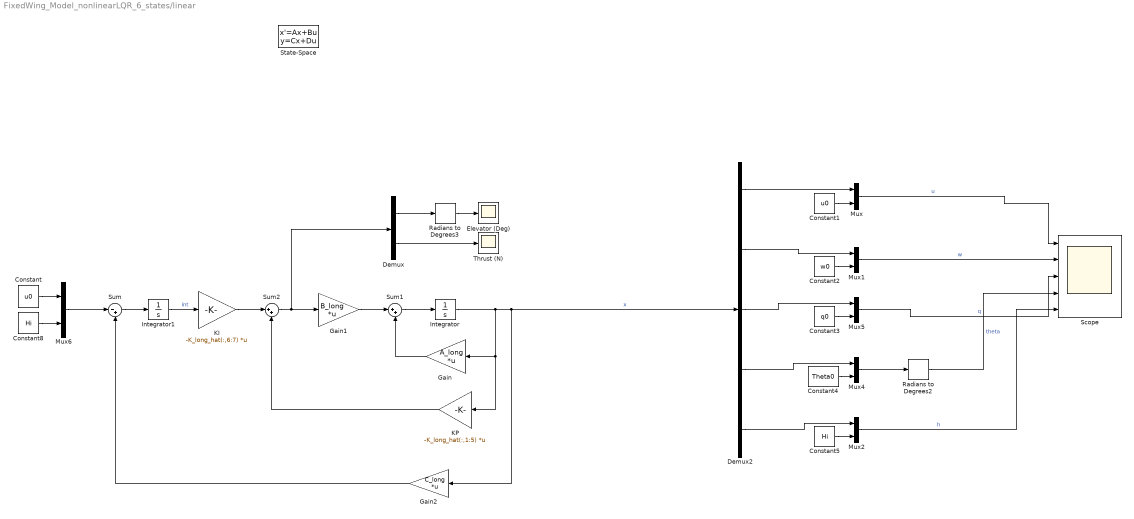
== system FixedWing_Model_nonlinearLQR_6_states/linear ==
  Constant : Constant  Value=u0
  Constant1 : Constant  Value=u0
  Constant2 : Constant  Value=w0
  Constant3 : Constant  Value=q0
  Constant4 : Constant  Value=Theta0
  Constant5 : Constant  Value=Hi
  Constant8 : Constant  Value=Hi
  Demux : Demux  Outputs=2
  Demux2 : Demux  Outputs=5
  Elevator (Deg) : Scope
  Gain : Gain  Gain=A_long  Multiplication=Matrix(K*u)
  Gain1 : Gain  Gain=B_long  Multiplication=Matrix(K*u)
  Gain2 : Gain  Gain=C_long  Multiplication=Matrix(K*u)
  Integrator : Integrator  InitialCondition=longi(1:5,:)
  Integrator1 : Integrator
  KI : Gain  Gain=-K_long_hat(:,6:7)  Multiplication=Matrix(K*u)
  KP : Gain  Gain=-K_long_hat(:,1:5)  Multiplication=Matrix(K*u)
  Mux{,1..2,4..6} (6 alike) : Mux  Inputs=2
  Radians to Degrees2 : simulink_extras/Transformations/Radians to Degrees
  Radians to Degrees3 : simulink_extras/Transformations/Radians to Degrees
  Scope : Scope  NumInputPorts=5
  State-Space : StateSpace  InitialCondition=0
  Sum : Sum  Inputs=|-+
  Sum1 : Sum  Inputs=|++
  Sum2 : Sum  Inputs=|++
  Thrust (N) : Scope
  wires:
  Sum1/1 -> Integrator/1
  Integrator/1 -> Demux2/1, Gain2/1, Gain/1, KP/1  "x"
  Gain/1 -> Sum1/2
  Gain1/1 -> Sum1/1
  Radians to Degrees2/1 -> Scope/4  "theta"
  Demux/1 -> Radians to Degrees3/1
  Radians to Degrees3/1 -> Elevator (Deg)/1
  Demux/2 -> Thrust (N)/1
  Mux/1 -> Scope/1  "u"
  Mux1/1 -> Scope/2  "w"
  Mux5/1 -> Scope/3  "q"
  Mux4/1 -> Radians to Degrees2/1
  Mux2/1 -> Scope/5  "h"
  Constant1/1 -> Mux/2
  Demux2/1 -> Mux/1
  Constant2/1 -> Mux1/2
  Constant3/1 -> Mux5/2
  Constant4/1 -> Mux4/2
  Constant5/1 -> Mux2/2
  Demux2/5 -> Mux2/1
  Demux2/4 -> Mux4/1
  Demux2/2 -> Mux1/1
  Demux2/3 -> Mux5/1
  Sum2/1 -> Demux/1, Gain1/1
  KP/1 -> Sum2/2
  Constant/1 -> Mux6/1
  Constant8/1 -> Mux6/2
  Sum/1 -> Integrator1/1
  KI/1 -> Sum2/1
  Mux6/1 -> Sum/1
  Gain2/1 -> Sum/2
  Integrator1/1 -> KI/1  "int"

== system FixedWing_Model_nonlinearLQR_6_states/linear dina 4 ==
  Constant : Constant  Value=longd
  Demux : Demux  Outputs=2
  Demux2 : Demux  Outputs=5
  Display : Display
  Elevator (Deg) : Scope
  Gain : Gain  Gain=A_hat  Multiplication=Matrix(K*u)
  Gain1 : Gain  Gain=B_hat  Multiplication=Matrix(K*u)
  Gain2 : Gain  Gain=C_hat  Multiplication=Matrix(K*u)
  Integrator : Integrator  InitialCondition=e_longi
  K_LQR1 : Gain  Gain=-K_long_hat  Multiplication=Matrix(K*u)
  Pitch Angle (Deg) : Scope
  Radians to Degrees1 : simulink_extras/Transformations/Radians to Degrees
  Radians to Degrees2 : simulink_extras/Transformations/Radians to Degrees
  Radians to Degrees3 : simulink_extras/Transformations/Radians to Degrees
  Sum1 : Sum  Inputs=|++
  Sum2 : Sum  Inputs=|-+
  Thrust (N) : Scope
  error pitch Angle (Deg) : Scope
  q : Scope
  u : Scope
  w : Scope
  wires:
  Sum1/1 -> Integrator/1
  Integrator/1 -> Gain2/1, Gain/1  "x"
  Gain/1 -> Sum1/2
  Gain1/1 -> Sum1/1
  K_LQR1/1 -> Gain1/1, Demux/1  "u"
  Gain2/1 -> Display/1, Sum2/1, K_LQR1/1  "y"
  Radians to Degrees2/1 -> Pitch Angle (Deg)/1
  Demux2/1 -> u/1
  Demux2/2 -> w/1
  Demux2/3 -> q/1
  Demux2/4 -> Radians to Degrees2/1
  Radians to Degrees1/1 -> error pitch Angle (Deg)/1
  Demux2/5 -> Radians to Degrees1/1
  Sum2/1 -> Demux2/1
  Constant/1 -> Sum2/2
  Demux/1 -> Radians to Degrees3/1
  Radians to Degrees3/1 -> Elevator (Deg)/1
  Demux/2 -> Thrust (N)/1

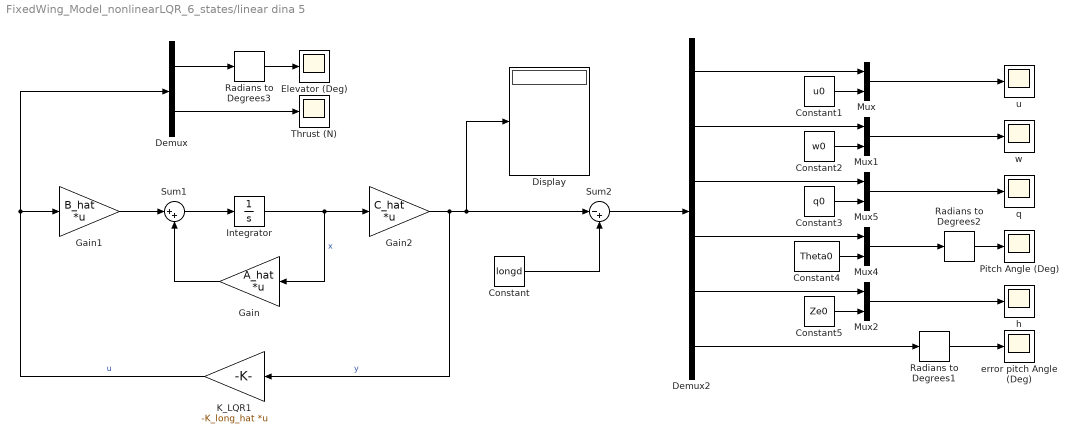
== system FixedWing_Model_nonlinearLQR_6_states/linear dina 5 ==
  Constant : Constant  Value=longd
  Constant1 : Constant  Value=u0
  Constant2 : Constant  Value=w0
  Constant3 : Constant  Value=q0
  Constant4 : Constant  Value=Theta0
  Constant5 : Constant  Value=Ze0
  Demux : Demux  Outputs=2
  Demux2 : Demux  Outputs=6
  Display : Display
  Elevator (Deg) : Scope
  Gain : Gain  Gain=A_hat  Multiplication=Matrix(K*u)
  Gain1 : Gain  Gain=B_hat  Multiplication=Matrix(K*u)
  Gain2 : Gain  Gain=C_hat  Multiplication=Matrix(K*u)
  Integrator : Integrator  InitialCondition=e_longi
  K_LQR1 : Gain  Gain=-K_long_hat  Multiplication=Matrix(K*u)
  Mux{,1..2,4..5} (5 alike) : Mux  Inputs=2
  Pitch Angle (Deg) : Scope
  Radians to Degrees1 : simulink_extras/Transformations/Radians to Degrees
  Radians to Degrees2 : simulink_extras/Transformations/Radians to Degrees
  Radians to Degrees3 : simulink_extras/Transformations/Radians to Degrees
  Sum1 : Sum  Inputs=|++
  Sum2 : Sum  Inputs=|-+
  Thrust (N) : Scope
  error pitch Angle (Deg) : Scope
  h : Scope
  q : Scope
  u : Scope
  w : Scope
  wires:
  Sum1/1 -> Integrator/1
  Integrator/1 -> Gain2/1, Gain/1  "x"
  Gain/1 -> Sum1/2
  Gain1/1 -> Sum1/1
  K_LQR1/1 -> Gain1/1, Demux/1  "u"
  Gain2/1 -> Display/1, Sum2/1, K_LQR1/1  "y"
  Radians to Degrees2/1 -> Pitch Angle (Deg)/1
  Radians to Degrees1/1 -> error pitch Angle (Deg)/1
  Sum2/1 -> Demux2/1
  Constant/1 -> Sum2/2
  Demux/1 -> Radians to Degrees3/1
  Radians to Degrees3/1 -> Elevator (Deg)/1
  Demux/2 -> Thrust (N)/1
  Demux2/6 -> Radians to Degrees1/1
  Mux/1 -> u/1
  Mux1/1 -> w/1
  Mux5/1 -> q/1
  Mux4/1 -> Radians to Degrees2/1
  Mux2/1 -> h/1
  Constant1/1 -> Mux/2
  Demux2/1 -> Mux/1
  Constant2/1 -> Mux1/2
  Constant3/1 -> Mux5/2
  Constant4/1 -> Mux4/2
  Constant5/1 -> Mux2/2
  Demux2/5 -> Mux2/1
  Demux2/4 -> Mux4/1
  Demux2/2 -> Mux1/1
  Demux2/3 -> Mux5/1

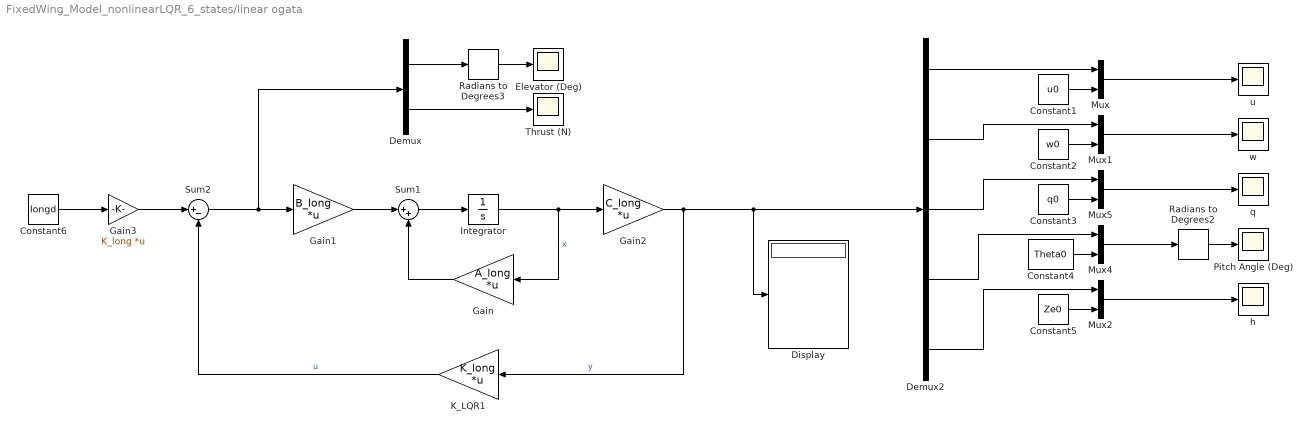
== system FixedWing_Model_nonlinearLQR_6_states/linear ogata ==
  Constant1 : Constant  Value=u0
  Constant2 : Constant  Value=w0
  Constant3 : Constant  Value=q0
  Constant4 : Constant  Value=Theta0
  Constant5 : Constant  Value=Ze0
  Constant6 : Constant  Value=longd
  Demux : Demux  Outputs=2
  Demux2 : Demux  Outputs=5
  Display : Display
  Elevator (Deg) : Scope
  Gain : Gain  Gain=A_long  Multiplication=Matrix(K*u)
  Gain1 : Gain  Gain=B_long  Multiplication=Matrix(K*u)
  Gain2 : Gain  Gain=C_long  Multiplication=Matrix(K*u)
  Gain3 : Gain  Gain=K_long  Multiplication=Matrix(K*u)
  Integrator : Integrator  InitialCondition=longi
  K_LQR1 : Gain  Gain=K_long  Multiplication=Matrix(K*u)
  Mux{,1..2,4..5} (5 alike) : Mux  Inputs=2
  Pitch Angle (Deg) : Scope
  Radians to Degrees2 : simulink_extras/Transformations/Radians to Degrees
  Radians to Degrees3 : simulink_extras/Transformations/Radians to Degrees
  Sum1 : Sum  Inputs=|++
  Sum2 : Sum  Inputs=|+-
  Thrust (N) : Scope
  h : Scope
  q : Scope
  u : Scope
  w : Scope
  wires:
  Sum1/1 -> Integrator/1
  Integrator/1 -> Gain/1, Gain2/1  "x"
  Gain/1 -> Sum1/2
  Gain1/1 -> Sum1/1
  K_LQR1/1 -> Sum2/2  "u"
  Gain2/1 -> K_LQR1/1, Display/1, Demux2/1  "y"
  Radians to Degrees2/1 -> Pitch Angle (Deg)/1
  Demux/1 -> Radians to Degrees3/1
  Radians to Degrees3/1 -> Elevator (Deg)/1
  Demux/2 -> Thrust (N)/1
  Mux/1 -> u/1
  Mux1/1 -> w/1
  Mux5/1 -> q/1
  Mux4/1 -> Radians to Degrees2/1
  Mux2/1 -> h/1
  Constant1/1 -> Mux/2
  Demux2/1 -> Mux/1
  Constant2/1 -> Mux1/2
  Constant3/1 -> Mux5/2
  Constant4/1 -> Mux4/2
  Constant5/1 -> Mux2/2
  Demux2/5 -> Mux2/1
  Demux2/4 -> Mux4/1
  Demux2/2 -> Mux1/1
  Demux2/3 -> Mux5/1
  Sum2/1 -> Demux/1, Gain1/1
  Constant6/1 -> Gain3/1
  Gain3/1 -> Sum2/1

== system FixedWing_Model_nonlinearLQR_6_states/linear paper ==
  Demux2 : Demux
  Gain : Gain  Gain=A_long  Multiplication=Matrix(K*u)
  Gain1 : Gain  Gain=B_long  Multiplication=Matrix(K*u)
  Gain2 : Gain  Gain=C_long  Multiplication=Matrix(K*u)
  Integrator : Integrator  InitialCondition=longi
  Integrator2 : Integrator  InitialCondition=[0 0 0 2*pi/180]
  K_LQR1 : Gain  Gain=-use  Multiplication=Matrix(K*u)
  Pitch Angle (Deg)1 : Scope
  Radians to Degrees2 : simulink_extras/Transformations/Radians to Degrees
  Sum1 : Sum  Inputs=|++
  q : Scope
  states' error1 : Subsystem
  u : Scope
  w : Scope
  wires:
  Sum1/1 -> Integrator/1
  Integrator/1 -> Gain2/1, Gain/1  "x"
  Gain/1 -> Sum1/2
  Gain1/1 -> Sum1/1
  K_LQR1/1 -> Gain1/1
  Gain2/1 -> states' error1/1(In1), Demux2/1  "y"
  Demux2/4 -> Radians to Degrees2/1
  Radians to Degrees2/1 -> Pitch Angle (Deg)1/1
  states' error1/1(states' error) -> Integrator2/1
  Demux2/1 -> u/1
  Demux2/2 -> w/1
  Demux2/3 -> q/1
  Integrator2/1 -> K_LQR1/1

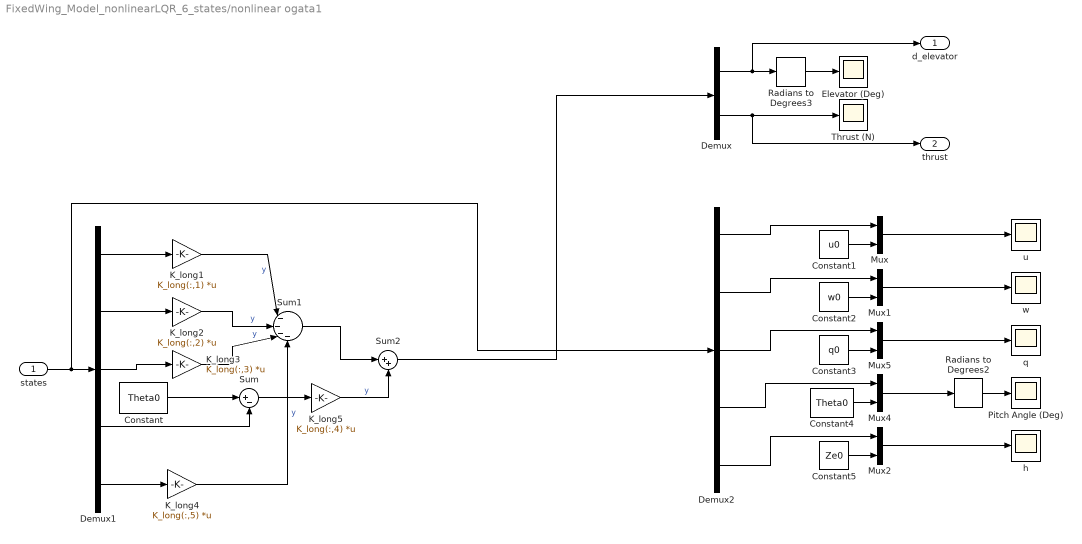
== system FixedWing_Model_nonlinearLQR_6_states/nonlinear ogata1 ==
  states : Inport
  Constant : Constant  Value=Theta0
  Constant1 : Constant  Value=u0
  Constant2 : Constant  Value=w0
  Constant3 : Constant  Value=q0
  Constant4 : Constant  Value=Theta0
  Constant5 : Constant  Value=Ze0
  Demux : Demux  Outputs=2
  Demux1 : Demux  Outputs=5
  Demux2 : Demux  Outputs=5
  Elevator (Deg) : Scope
  K_long1 : Gain  Gain=K_long(:,1)  Multiplication=Matrix(K*u)
  K_long2 : Gain  Gain=K_long(:,2)  Multiplication=Matrix(K*u)
  K_long3 : Gain  Gain=K_long(:,3)  Multiplication=Matrix(K*u)
  K_long4 : Gain  Gain=K_long(:,5)  Multiplication=Matrix(K*u)
  K_long5 : Gain  Gain=K_long(:,4)  Multiplication=Matrix(K*u)
  Mux{,1..2,4..5} (5 alike) : Mux  Inputs=2
  Pitch Angle (Deg) : Scope
  Radians to Degrees2 : simulink_extras/Transformations/Radians to Degrees
  Radians to Degrees3 : simulink_extras/Transformations/Radians to Degrees
  Sum : Sum  Inputs=|+-
  Sum1 : Sum  Inputs=|----
  Sum2 : Sum  Inputs=|++
  Thrust (N) : Scope
  h : Scope
  q : Scope
  u : Scope
  w : Scope
  d_elevator : Outport
  thrust : Outport  Port=2
  wires:
  Radians to Degrees2/1 -> Pitch Angle (Deg)/1
  Demux/1 -> d_elevator/1, Radians to Degrees3/1
  Radians to Degrees3/1 -> Elevator (Deg)/1
  Demux/2 -> Thrust (N)/1, thrust/1
  Mux/1 -> u/1
  Mux1/1 -> w/1
  Mux5/1 -> q/1
  Mux4/1 -> Radians to Degrees2/1
  Mux2/1 -> h/1
  Constant1/1 -> Mux/2
  Demux2/1 -> Mux/1
  Constant2/1 -> Mux1/2
  Constant3/1 -> Mux5/2
  Constant4/1 -> Mux4/2
  Constant5/1 -> Mux2/2
  Demux2/5 -> Mux2/1
  Demux2/4 -> Mux4/1
  Demux2/2 -> Mux1/1
  Demux2/3 -> Mux5/1
  states/1 -> Demux2/1, Demux1/1
  K_long1/1 -> Sum1/1  "y"
  K_long2/1 -> Sum1/2  "y"
  K_long3/1 -> Sum1/3  "y"
  K_long4/1 -> Sum1/4  "y"
  Demux1/5 -> K_long4/1
  Demux1/3 -> K_long3/1
  Demux1/2 -> K_long2/1
  Demux1/1 -> K_long1/1
  Demux1/4 -> Sum/2
  Constant/1 -> Sum/1
  Sum1/1 -> Sum2/1
  Sum/1 -> K_long5/1
  Sum2/1 -> Demux/1
  K_long5/1 -> Sum2/2  "y"

== system FixedWing_Model_nonlinearLQR_6_states/Aerodynamic /Delta L moment ==
  v : Inport
  p : Inport  Port=2
  r : Inport  Port=3
  rudder : Inport  Port=4
  Q : Inport  Port=5
  aileron : Inport  Port=6
  Add : Sum  Inputs=+++++
  Subsystem : Subsystem
  Subsystem1 : Subsystem
  Subsystem2 : Subsystem
  Subsystem3 : Subsystem
  Subsystem4 : Subsystem
  Out1 : Outport
  wires:
  Subsystem4/1(Out1) -> Add/1
  Subsystem3/1(Out1) -> Add/2
  Subsystem/1(Out1) -> Add/3
  Subsystem1/1(Out1) -> Add/4
  Subsystem2/1(Out1) -> Add/5
  Add/1 -> Out1/1
  v/1 -> Subsystem4/1(v)
  p/1 -> Subsystem3/1(p)
  r/1 -> Subsystem/1(r)
  rudder/1 -> Subsystem1/1(rudder)
  aileron/1 -> Subsystem2/1(aileron)
  Q/1 -> [Q]
  [Q] -> Subsystem4/2(Q)
  [Q] -> Subsystem3/2(Q)
  [Q] -> Subsystem/2(Q)
  [Q] -> Subsystem1/2(Q)
  [Q] -> Subsystem2/2(Q)

== system FixedWing_Model_nonlinearLQR_6_states/Aerodynamic /Delta M moment ==
  u : Inport
  w : Inport  Port=2
  w_dot : Inport  Port=3
  q : Inport  Port=4
  elevator : Inport  Port=5
  Thrust : Inport  Port=6
  Q : Inport  Port=7
  Add : Sum  Inputs=++++++
  Subsystem : Subsystem
  Subsystem1 : Subsystem
  Subsystem2 : Subsystem
  Subsystem3 : Subsystem
  Subsystem4 : Subsystem
  Subsystem5 : Subsystem
  Out1 : Outport
  wires:
  Subsystem1/1(Out1) -> Add/4
  Subsystem4/1(Out1) -> Add/1
  w/1 -> Subsystem3/1(w)
  w_dot/1 -> Subsystem/1(w_dot)
  Subsystem3/1(Out1) -> Add/2
  q/1 -> Subsystem1/1(q)
  Subsystem/1(Out1) -> Add/3
  Add/1 -> Out1/1
  u/1 -> Subsystem4/1(u)
  Subsystem5/1(Out1) -> Add/6
  Thrust/1 -> Subsystem5/1(Thrust)
  Q/1 -> [Q]
  [Q] -> Subsystem4/2(Q)
  [Q] -> Subsystem3/2(Q)
  [Q] -> Subsystem/2(Q)
  [Q] -> Subsystem1/2(Q)
  Subsystem2/1(Out3) -> Add/5
  [Q] -> Subsystem2/2(Q)
  elevator/1 -> Subsystem2/1(elevator)
  [Q] -> Subsystem5/2(Q)

== system FixedWing_Model_nonlinearLQR_6_states/Aerodynamic /Delta N moment ==
  v : Inport
  p : Inport  Port=2
  r : Inport  Port=3
  rudder : Inport  Port=4
  aileron : Inport  Port=5
  Q : Inport  Port=6
  Add : Sum  Inputs=+++++
  Subsystem : Subsystem
  Subsystem1 : Subsystem
  Subsystem2 : Subsystem
  Subsystem3 : Subsystem
  Subsystem4 : Subsystem
  Out1 : Outport
  wires:
  rudder/1 -> Subsystem1/1(rudder)
  p/1 -> Subsystem3/1(p)
  Subsystem/1(Out1) -> Add/3
  Subsystem3/1(Out1) -> Add/2
  r/1 -> Subsystem/1(r)
  Subsystem2/1(Out1) -> Add/5
  Subsystem1/1(Out1) -> Add/4
  Subsystem4/1(Out1) -> Add/1
  aileron/1 -> Subsystem2/1(aileron)
  Add/1 -> Out1/1
  v/1 -> Subsystem4/1(v)
  Q/1 -> [Q]
  [Q] -> Subsystem4/2(Q)
  [Q] -> Subsystem3/2(Q)
  [Q] -> Subsystem/2(Q)
  [Q] -> Subsystem1/2(Q)
  [Q] -> Subsystem2/2(Q)

== system FixedWing_Model_nonlinearLQR_6_states/Aerodynamic /Delta X force ==
  u : Inport
  w : Inport  Port=2
  Q : Inport  Port=3
  elevator : Inport  Port=4
  Thrust : Inport  Port=5
  Add : Sum  Inputs=++++
  Display{,1..3} (4 alike) : Display
  Subsystem : Subsystem
  Subsystem1 : Subsystem
  Subsystem2 : Subsystem
  Subsystem3 : Subsystem
  delta X force : Outport
  wires:
  Add/1 -> delta X force/1
  Subsystem/1(Out1) -> Display/1, Add/1
  Subsystem2/1(Out1) -> Display2/1, Add/3
  Subsystem1/1(Out1) -> Display1/1, Add/2
  Q/1 -> [Q]
  [Q] -> Subsystem/1(Q)
  [Q] -> Subsystem1/1(Q)
  [Q] -> Subsystem2/1(Q)
  [Q] -> Subsystem3/1(Q)
  Subsystem3/1(Out2) -> Display3/1, Add/4
  w/1 -> Subsystem1/2(w)
  elevator/1 -> Subsystem2/2(elevator)  "delta_elevator"
  Thrust/1 -> Subsystem3/2(Thrust)  "Delta_thrust"
  u/1 -> Subsystem/2(u)

== system FixedWing_Model_nonlinearLQR_6_states/Aerodynamic /Delta Z force ==
  w_dot : Inport
  u : Inport  Port=2
  Q : Inport  Port=3
  w : Inport  Port=4
  q : Inport  Port=5
  elevator : Inport  Port=6
  Thrust : Inport  Port=7
  Add : Sum  Inputs=++++++
  Display{,1..5} (6 alike) : Display
  Subsystem : Subsystem
  Subsystem1 : Subsystem
  Subsystem2 : Subsystem
  Subsystem3 : Subsystem
  Subsystem4 : Subsystem
  Subsystem6 : Subsystem
  delta Z force : Outport
  wires:
  u/1 -> Subsystem4/1(u)
  Add/1 -> delta Z force/1
  Subsystem2/1(Out1) -> Display3/1, Add/4
  Subsystem3/1(Out1) -> Display4/1, Add/5
  Subsystem6/1(Out1) -> Display5/1, Add/6
  Subsystem4/1(Out2) -> Display/1, Add/1
  Q/1 -> [Q]
  [Q] -> Subsystem4/2(Q)
  w/1 -> Subsystem/1(w)
  [Q] -> Subsystem/2(Q)
  Subsystem/1(Out2) -> Add/2, Display1/1
  w_dot/1 -> Subsystem1/1(w_dot)
  [Q] -> Subsystem1/2(Q)
  Subsystem1/1(Out2) -> Display2/1, Add/3
  q/1 -> Subsystem2/1(q)
  [Q] -> Subsystem2/2(Q)
  elevator/1 -> Subsystem3/1(elevator)
  [Q] -> Subsystem3/2(Q)
  Thrust/1 -> Subsystem6/1(Thrust)
  [Q] -> Subsystem6/2(Q)

== system FixedWing_Model_nonlinearLQR_6_states/Aerodynamic /DeltaY force ==
  v : Inport
  p : Inport  Port=2
  r : Inport  Port=3
  Q : Inport  Port=4
  rudder : Inport  Port=5
  Add : Sum  Inputs=++++
  Subsystem : Subsystem
  Subsystem1 : Subsystem
  Subsystem2 : Subsystem
  Subsystem3 : Subsystem
  delta Y force : Outport
  wires:
  Subsystem3/1(Out1) -> Add/4
  Subsystem/1(Out1) -> Add/1
  Add/1 -> delta Y force/1
  v/1 -> Subsystem/1(v)
  p/1 -> Subsystem1/1(p)
  r/1 -> Subsystem2/1(r)
  rudder/1 -> Subsystem3/1(rudder)
  Q/1 -> [Q]
  [Q] -> Subsystem/2(Q)
  Subsystem1/1(Out2) -> Add/2
  [Q] -> Subsystem1/2(Q)
  [Q] -> Subsystem2/2(Q)
  Subsystem2/1(Out2) -> Add/3
  [Q] -> Subsystem3/2(Q)

== system FixedWing_Model_nonlinearLQR_6_states/Longitudinal LQR elevator &thrust/all system ==
  states : Inport
  Actual theta : Scope
  Constant1 : Constant  Value=d_elevator0
  Constant2 : Constant  Value=d_Thrust0
  Demux : Demux  Outputs=2
  Gain1 : Gain
  Gain2 : Gain
  K_LQR : Gain  Gain=K_long  Multiplication=Matrix(K*u)
  Radians to Degrees4 : simulink_extras/Transformations/Radians to Degrees
  Sum1 : Sum  Inputs=|++
  Sum2 : Sum  Inputs=|++
  Thrust : Scope
  elevator2 : Scope
  states' error : Subsystem
  d_elevator : Outport
  thrust : Outport  Port=2
  wires:
  states' error/1(theta in degrees) -> Actual theta/1
  states/1 -> states' error/1(In1)
  states' error/2(states' error) -> K_LQR/1
  Constant1/1 -> Sum1/2
  K_LQR/1 -> Demux/1
  Sum1/1 -> Gain2/1, Radians to Degrees4/1
  Gain2/1 -> d_elevator/1  "d_elevator"
  Radians to Degrees4/1 -> elevator2/1
  Demux/1 -> Sum1/1
  Gain1/1 -> thrust/1  "thrust"
  Demux/2 -> Sum2/1
  Constant2/1 -> Sum2/2
  Sum2/1 -> Thrust/1, Gain1/1

== system FixedWing_Model_nonlinearLQR_6_states/Longitudinal LQR elevator only/all system ==
  states : Inport
  Actual theta1 : Scope
  Constant1 : Constant  Value=d_elevator0
  Gain2 : Gain
  K_LQR1 : Gain  Gain=K_long  Multiplication=Matrix(K*u)
  Radians to Degrees4 : simulink_extras/Transformations/Radians to Degrees
  Sum1 : Sum  Inputs=|++
  elevator2 : Scope
  states' error : Subsystem
  d_elevator : Outport
  wires:
  states' error/1(theta in degrees) -> Actual theta1/1
  states/1 -> states' error/1(In1)
  states' error/2(states' error) -> K_LQR1/1
  Constant1/1 -> Sum1/2
  K_LQR1/1 -> Sum1/1
  Sum1/1 -> Gain2/1, Radians to Degrees4/1
  Gain2/1 -> d_elevator/1  "d_elevator"
  Radians to Degrees4/1 -> elevator2/1

== system FixedWing_Model_nonlinearLQR_6_states/Longitudinal LQR elevator only/states from ss ==
  Demux : Demux  Commented=on
  Gain1 : Gain  Commented=on
  K_LQR2 : Gain  Commented=on  Gain=K_long  Multiplication=Matrix(K*u)
  Radians to Degrees2 : simulink_extras/Transformations/Radians to Degrees  Commented=on
  State-Space1 : StateSpace  Commented=on  A=A_long  B=B_long  C=C_long  D=D_long  InitialCondition=longi
  Sum1 : Sum  Inputs=|+-
  Theta LQR1 : Scope  Commented=on
  elevator1 : Scope  Commented=on
  states' error : Subsystem  Commented=on
  elevator demand1 : Outport
  wires:
  Radians to Degrees2/1 -> elevator1/1
  Sum1/1 -> State-Space1/1  "u"
  states' error/2(states' error) -> Demux/1, K_LQR2/1
  Demux/4 -> Sum1/1, Radians to Degrees2/1, Gain1/1
  State-Space1/1 -> states' error/1(In1)  "y"
  K_LQR2/1 -> Sum1/2
  states' error/1(theta in degrees) -> Theta LQR1/1
  Gain1/1 -> elevator demand1/1  "d_elevator"

== system FixedWing_Model_nonlinearLQR_6_states/Longitudinal LQR elevator only/theta from ss ==
  Constant : Constant  Commented=on  Value=Theta0
  Constant1 : Constant  Commented=on  Value=d_elevator0
  Demux7 : Demux  Commented=on
  Gain3 : Gain  Commented=on
  K_LQR1 : Gain  Commented=on  Gain=K_long(1,4)  Multiplication=Matrix(K*u)
  Radians to Degrees1 : simulink_extras/Transformations/Radians to Degrees  Commented=on
  Radians to Degrees3 : simulink_extras/Transformations/Radians to Degrees  Commented=on
  State-Space3 : StateSpace  Commented=on  A=A_long  B=B_long  C=C_long  D=D_long  InitialCondition=longi
  Sum7 : Sum  Commented=on  Inputs=|+-
  Sum8 : Sum  Commented=on  Inputs=|+-
  Theta LQR : Scope  Commented=on
  elevator : Scope  Commented=on
  elevator demand : Outport
  wires:
  Radians to Degrees3/1 -> elevator/1
  Sum8/1 -> K_LQR1/1, Gain3/1, Radians to Degrees3/1  "error theta"
  K_LQR1/1 -> Sum7/2
  Radians to Degrees1/1 -> Theta LQR/1
  State-Space3/1 -> Demux7/1  "y"
  Constant/1 -> Sum8/2
  Demux7/4 -> Sum8/1, Radians to Degrees1/1
  Constant1/1 -> Sum7/1
  Sum7/1 -> State-Space3/1  "u"
  Gain3/1 -> elevator demand/1  "d_elevator"

== system FixedWing_Model_nonlinearLQR_6_states/Longitudinal LQR elevator only/theta system only ==
  theta : Inport
  Actual theta1 : Scope
  Constant2 : Constant  Value=d_elevator0
  Constant3 : Constant  Value=Theta0
  Gain2 : Gain
  K_LQR3 : Gain  Gain=K_long(1,4)  Multiplication=Matrix(K*u)
  Radians to Degrees4 : simulink_extras/Transformations/Radians to Degrees
  Radians to Degrees5 : simulink_extras/Transformations/Radians to Degrees
  Sum2 : Sum  Inputs=|+-
  Sum3 : Sum  Inputs=|+-
  elevator2 : Scope
  d_elevator : Outport
  wires:
  Radians to Degrees4/1 -> elevator2/1
  Sum3/1 -> K_LQR3/1  "error theta"
  theta/1 -> Radians to Degrees5/1, Sum3/1
  K_LQR3/1 -> Sum2/2
  Constant3/1 -> Sum3/2
  Radians to Degrees5/1 -> Actual theta1/1
  Gain2/1 -> d_elevator/1  "d_elevator"
  Constant2/1 -> Sum2/1
  Sum2/1 -> Gain2/1, Radians to Degrees4/1
